simulink model "EsamblajeCohete2_0"  (R2023a)
settings: Solver=VariableStepAuto  StartTime=0.0  StopTime=120  RelTol=1e-3
model workspace: external: MATLAB File C:\Users\SEBASTIANDIAZPABON\OneDrive - Universidad Santo Tomás Bucaramanga\USTA\Semillero Cohete\Cohete Matlab 2.0\EsamblajeCohete2_0_DataFile.m (data not in the file)
undefined symbols (not defined in the file): smiData, X, Y, Z
libraries: sm_lib x354, nesl_utility x13, simulink x7, fuzblock x6
(part 1 of 7)
settings Model: SimulationMode=accelerator  Creator=SEBASTIANDIAZPABON  LastModifiedBy=SEBASTIANDIAZPABON
settings ModelReferenceCC: EnableRefExpFcnMdlSchedulingChecks=on

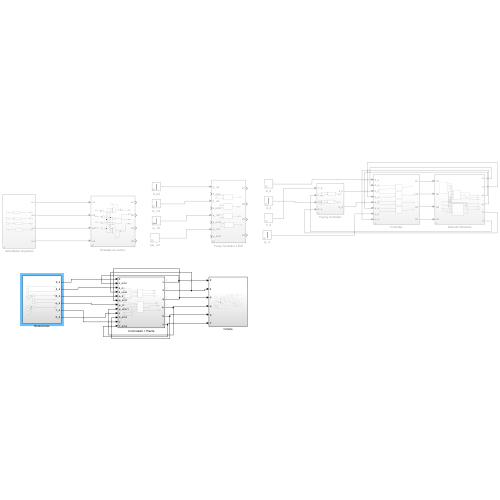
[thumbnail: Simulink's stored preview of the top-level diagram]
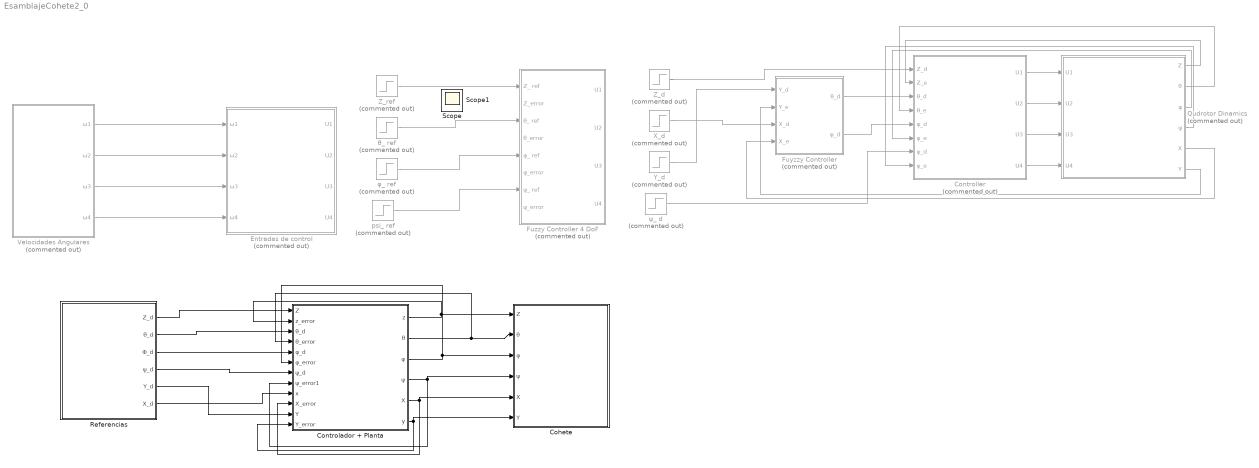
== system EsamblajeCohete2_0 ==
  Cohete : Subsystem
  Controlador + Planta : Subsystem
  Controller : Subsystem  Commented=on
  "Entradas de control " : Subsystem  Commented=on
  Fuyzzy Controller : Subsystem  Commented=on
  Fuzzy Controller 4 DoF : Subsystem  Commented=on
  Qudrotor Dinamics : Subsystem  Commented=on
  Referencias : Subsystem
  Velocidades Angulares : Subsystem  Commented=on
  X_d : Step  Commented=on  After=20  SampleTime=0
  Y_d : Step  Commented=on  After=20  SampleTime=0
  Z_d : Step  Commented=on  Time=0.01  After=30  SampleTime=0
  Z_ref : Step  Commented=on  Time=0  After=0  SampleTime=0
  psi_ ref : Step  Commented=on  Time=0  After=0.05  SampleTime=0
  θ_ ref : Step  Commented=on  Time=0  After=0.1  SampleTime=0
  φ_ ref : Step  Commented=on  Time=0  After=0.5  SampleTime=0
  ψ_ d : Step  Commented=on  After=20  SampleTime=0
  Scope : Scope
  Scope1 : Scope
  wires:
  Velocidades Angulares/1(ω1) -> "Entradas de control "/1(ω1)
  Velocidades Angulares/2(ω2) -> "Entradas de control "/2(ω2)
  Velocidades Angulares/3(ω3) -> "Entradas de control "/3(ω3)
  Velocidades Angulares/4(ω4) -> "Entradas de control "/4(ω4)
  Z_ref/1 -> Fuzzy Controller 4 DoF/1(Z_ ref)
  θ_ ref/1 -> Fuzzy Controller 4 DoF/3(θ_ ref)
  φ_ ref/1 -> Fuzzy Controller 4 DoF/5(φ_ ref)
  psi_ ref/1 -> Fuzzy Controller 4 DoF/7(ψ_ ref)
  Controller/1(U1) -> Qudrotor Dinamics/1(U1)
  Controller/2(U2) -> Qudrotor Dinamics/2(U2)
  Controller/3(U3) -> Qudrotor Dinamics/3(U3)
  Controller/4(U4) -> Qudrotor Dinamics/4(U4)
  Qudrotor Dinamics/1(Z) -> Controller/2(Z_e)
  Qudrotor Dinamics/2(θ) -> Controller/4(θ_e)
  Qudrotor Dinamics/3(φ) -> Controller/6(φ_e)
  Qudrotor Dinamics/4(ψ) -> Controller/8(ψ_e)
  Fuyzzy Controller/1(θ_d) -> Controller/3(θ_d)
  Qudrotor Dinamics/6(Y) -> Fuyzzy Controller/2(Y_e)
  Qudrotor Dinamics/5(X) -> Fuyzzy Controller/4(X_e)
  Fuyzzy Controller/2(φ_d) -> Controller/5(φ_d)
  Z_d/1 -> Controller/1(Z_d)
  X_d/1 -> Fuyzzy Controller/3(X_d)
  Y_d/1 -> Fuyzzy Controller/1(Y_d)
  ψ_ d/1 -> Controller/7(ψ_d)
  Controlador + Planta/1(z) -> Controlador + Planta/2(z_error), Cohete/1(Z)
  Referencias/1(Z_d) -> Controlador + Planta/1(Z)
  Controlador + Planta/2(θ) -> Controlador + Planta/4(θ_error), Cohete/2(θ)
  Controlador + Planta/3(φ) -> Cohete/3(φ), Controlador + Planta/6(φ_error)
  Controlador + Planta/4(ψ) -> Controlador + Planta/8(ψ_error1), Cohete/4(ψ)
  Referencias/2(θ_d) -> Controlador + Planta/3(θ_d)
  Referencias/4(ψ_d) -> Controlador + Planta/7(ψ_d)
  Referencias/3(Φ_d) -> Controlador + Planta/5(φ_d)
  Controlador + Planta/5(X) -> Controlador + Planta/10(X_error), Cohete/5(X)
  Referencias/6(X_d) -> Controlador + Planta/9(x)
  Controlador + Planta/6(y) -> Cohete/6(Y), Controlador + Planta/12(Y_error)
  Referencias/5(Y_d) -> Controlador + Planta/11(Y)

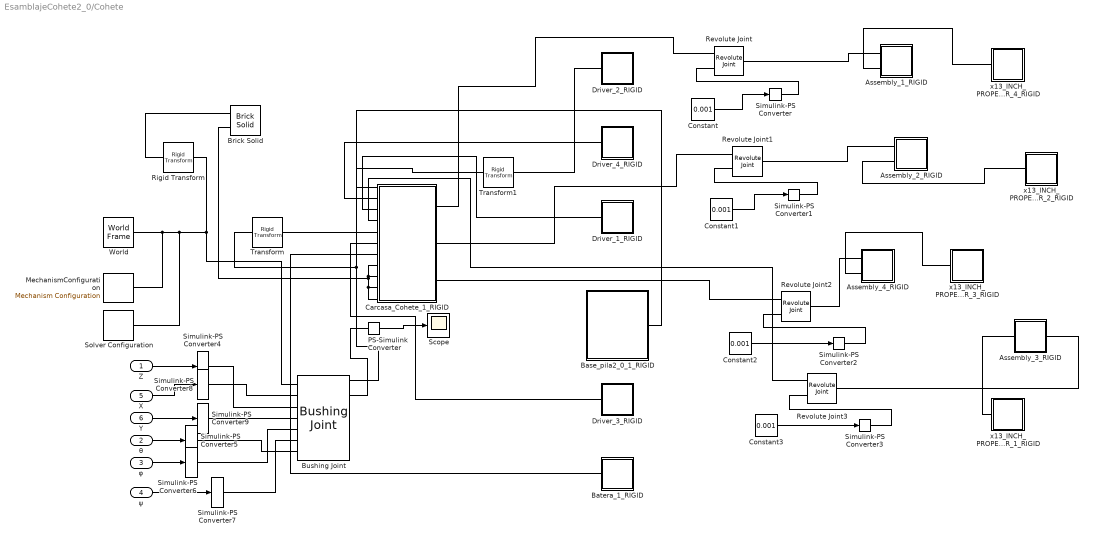
== system EsamblajeCohete2_0/Cohete ==
  Z : Inport
  θ : Inport  Port=2
  φ : Inport  Port=3
  ψ : Inport  Port=4
  X : Inport  Port=5
  Y : Inport  Port=6
  Assembly_1_RIGID : Subsystem
  Assembly_2_RIGID : Subsystem
  Assembly_3_RIGID : Subsystem
  Assembly_4_RIGID : Subsystem
  Base_pila2_0_1_RIGID : Subsystem
  Batera_1_RIGID : Subsystem
  Brick Solid : sm_lib/Body Elements/Brick Solid  GraphicAmbientColor=[0.15 0.15 0.15 1.0]  BasedOnType=Density  BrickDimensions=[2 2 0.1 ]  BrickDimensionsUnits=m  CenterOfMass=[0 0 0]  CenterOfMassUnits=m  GraphicDiffuseColor=[0.4 0.6 0.0]  Density=1000  DensityUnits=kg/m^3  DoExposeReferenceFrame=on  GraphicEmissiveColor=[0.0 0.0 0.0 1.0]  ExportEntireGeometry=on  SerializedFrames=<Frames><Frame><Id>Frame1</Id><Value><Name>F1</Name><Origin><Source>ReferenceFrame</Source><FeatureName></FeatureName></Origin><PrimaryAxis><DefinedDirection>+Y</DefinedDirection><Source>ReferenceFrame</Source><SourceDirection>-Z</SourceDirection><FeatureName></FeatureName></PrimaryAxis><SecondaryAxis><DefinedDirection>+X</DefinedDirection><Source>ReferenceFrame</Source><SourceDirection>+X</SourceDirection><FeatureName></FeatureName></SecondaryAxis></Value></Frame></Frames>  MarkerShape=Sphere  MarkerSize=10  GraphicType=FromGeometry  InertiaType=CalculateFromGeometry  Mass=1  MassUnits=kg  MomentsOfInertia=[1 1 1]  MomentsOfInertiaUnits=kg*m^2  GraphicOpacity=1.0  ProductsOfInertia=[0 0 0]  ProductsOfInertiaUnits=kg*m^2  GraphicShininess=75  GraphicSpecularColor=[0.5 0.5 0.5 1.0]  GraphicVisPropType=SimpleVisualProperties
  Bushing Joint : sm_lib/Joints/Bushing Joint  JointMode=Normal  SenseConstraintForce=off  SenseConstraintForceX=off  SenseConstraintForceY=off  SenseConstraintForceZ=off  SenseConstraintTorque=off  SenseConstraintTorqueX=off  SenseConstraintTorqueY=off  SenseConstraintTorqueZ=off  SenseTotalForce=off  SenseTotalForceX=off  SenseTotalForceY=off  SenseTotalForceZ=off  SenseTotalTorque=off  SenseTotalTorqueX=off  SenseTotalTorqueY=off  SenseTotalTorqueZ=off  CompositeWrenchDir=FollowerOnBase  CompositeWrenchFrame=BaseFrame  PxEquilibriumPosition=0  PxEquilibriumPositionUnits=m  PxSpringStiffness=0  PxSpringStiffnessUnits=N/m  PxDampingCoefficient=0  PxDampingCoefficientUnits=N/(m/s)  PxTorqueActuationMode=ComputedTorque  PxMotionActuationMode=InputMotion  PxSensePosition=off  PxSenseVelocity=off  PxSenseAcceleration=off  PxSenseTorqueForce=on  PxSenseLowerLimitTorqueForce=off  PxSenseUpperLimitTorqueForce=off  PxLowerLimitSpecify=off  PxLowerLimitBound=-1  PxLowerLimitBoundUnits=m  PxLowerLimitStiffness=1e6  PxLowerLimitStiffnessUnits=N/m  PxLowerLimitDamping=1e3  PxLowerLimitDampingUnits=N/(m/s)  PxLowerLimitTransitionRegionWidth=1e-4  PxLowerLimitTransitionRegionWidthUnits=m  PxUpperLimitSpecify=off  PxUpperLimitBound=1  PxUpperLimitBoundUnits=m  PxUpperLimitStiffness=1e6  PxUpperLimitStiffnessUnits=N/m  PxUpperLimitDamping=1e3  PxUpperLimitDampingUnits=N/(m/s)  PxUpperLimitTransitionRegionWidth=1e-4  PxUpperLimitTransitionRegionWidthUnits=m  PxPositionTargetSpecify=off  PxPositionTargetPriority=High  PxPositionTargetValue=0  PxPositionTargetValueUnits=m  PxVelocityTargetSpecify=off  PxVelocityTargetPriority=High  PxVelocityTargetValue=0  PxVelocityTargetValueUnits=m/s  PyEquilibriumPosition=0  PyEquilibriumPositionUnits=m  PySpringStiffness=0  PySpringStiffnessUnits=N/m  PyDampingCoefficient=0  PyDampingCoefficientUnits=N/(m/s)  PyTorqueActuationMode=ComputedTorque  PyMotionActuationMode=InputMotion  PySensePosition=on  PySenseVelocity=on  PySenseAcceleration=off  PySenseTorqueForce=off  PySenseLowerLimitTorqueForce=off  PySenseUpperLimitTorqueForce=off  PyLowerLimitSpecify=off  PyLowerLimitBound=-1  PyLowerLimitBoundUnits=m  PyLowerLimitStiffness=1e6  PyLowerLimitStiffnessUnits=N/m  PyLowerLimitDamping=1e3  PyLowerLimitDampingUnits=N/(m/s)  PyLowerLimitTransitionRegionWidth=1e-4  PyLowerLimitTransitionRegionWidthUnits=m  PyUpperLimitSpecify=off  PyUpperLimitBound=1  PyUpperLimitBoundUnits=m  PyUpperLimitStiffness=1e6  PyUpperLimitStiffnessUnits=N/m  PyUpperLimitDamping=1e3  PyUpperLimitDampingUnits=N/(m/s)  PyUpperLimitTransitionRegionWidth=1e-4  PyUpperLimitTransitionRegionWidthUnits=m  PyPositionTargetSpecify=off  PyPositionTargetPriority=High  PyPositionTargetValue=0  PyPositionTargetValueUnits=m  PyVelocityTargetSpecify=off  PyVelocityTargetPriority=High  PyVelocityTargetValue=0  PyVelocityTargetValueUnits=m/s  PzEquilibriumPosition=0  PzEquilibriumPositionUnits=m  PzSpringStiffness=0  PzSpringStiffnessUnits=N/m  PzDampingCoefficient=0  PzDampingCoefficientUnits=N/(m/s)  PzTorqueActuationMode=ComputedTorque  PzMotionActuationMode=InputMotion  PzSensePosition=off  PzSenseVelocity=off  PzSenseAcceleration=off  PzSenseTorqueForce=off  PzSenseLowerLimitTorqueForce=off  PzSenseUpperLimitTorqueForce=off  PzLowerLimitSpecify=off  PzLowerLimitBound=-1  PzLowerLimitBoundUnits=m  PzLowerLimitStiffness=1e6  PzLowerLimitStiffnessUnits=N/m  PzLowerLimitDamping=1e3  PzLowerLimitDampingUnits=N/(m/s)  PzLowerLimitTransitionRegionWidth=1e-4  PzLowerLimitTransitionRegionWidthUnits=m  PzUpperLimitSpecify=off  PzUpperLimitBound=1  PzUpperLimitBoundUnits=m  PzUpperLimitStiffness=1e6  PzUpperLimitStiffnessUnits=N/m  PzUpperLimitDamping=1e3  PzUpperLimitDampingUnits=N/(m/s)  PzUpperLimitTransitionRegionWidth=1e-4  PzUpperLimitTransitionRegionWidthUnits=m  PzPositionTargetSpecify=off  PzPositionTargetPriority=High  PzPositionTargetValue=0  PzPositionTargetValueUnits=m  PzVelocityTargetSpecify=off  PzVelocityTargetPriority=High  PzVelocityTargetValue=0  PzVelocityTargetValueUnits=m/s  RxEquilibriumPosition=0  RxEquilibriumPositionUnits=deg  RxSpringStiffness=0  RxSpringStiffnessUnits=N*m/deg  RxDampingCoefficient=0  RxDampingCoefficientUnits=N*m/(deg/s)  RxTorqueActuationMode=ComputedTorque  RxMotionActuationMode=InputMotion  RxSensePosition=on  RxSenseVelocity=on  RxSenseAcceleration=off  RxSenseTorqueForce=off  RxSenseLowerLimitTorqueForce=off  RxSenseUpperLimitTorqueForce=off  RxLowerLimitSpecify=off  RxLowerLimitBound=-90  RxLowerLimitBoundUnits=deg  RxLowerLimitStiffness=1e4  RxLowerLimitStiffnessUnits=N*m/deg  RxLowerLimitDamping=10  RxLowerLimitDampingUnits=N*m/(deg/s)  RxLowerLimitTransitionRegionWidth=0.1  RxLowerLimitTransitionRegionWidthUnits=deg  RxUpperLimitSpecify=off  RxUpperLimitBound=90  RxUpperLimitBoundUnits=deg  RxUpperLimitStiffness=1e4  RxUpperLimitStiffnessUnits=N*m/deg  RxUpperLimitDamping=10  RxUpperLimitDampingUnits=N*m/(deg/s)  RxUpperLimitTransitionRegionWidth=0.1  RxUpperLimitTransitionRegionWidthUnits=deg  RxPositionTargetSpecify=off  RxPositionTargetPriority=High  RxPositionTargetValue=0  RxPositionTargetValueUnits=deg  RxVelocityTargetSpecify=off  RxVelocityTargetPriority=High  RxVelocityTargetValue=0  RxVelocityTargetValueUnits=deg/s  RyEquilibriumPosition=0  RyEquilibriumPositionUnits=deg  RySpringStiffness=0  RySpringStiffnessUnits=N*m/deg  RyDampingCoefficient=0  RyDampingCoefficientUnits=N*m/(deg/s)  RyTorqueActuationMode=ComputedTorque  RyMotionActuationMode=InputMotion  RySensePosition=off  RySenseVelocity=off  RySenseAcceleration=off  RySenseTorqueForce=off  RySenseLowerLimitTorqueForce=off  RySenseUpperLimitTorqueForce=off  RyLowerLimitSpecify=off  RyLowerLimitBound=-90  RyLowerLimitBoundUnits=deg  RyLowerLimitStiffness=1e4  RyLowerLimitStiffnessUnits=N*m/deg  RyLowerLimitDamping=10  RyLowerLimitDampingUnits=N*m/(deg/s)  RyLowerLimitTransitionRegionWidth=0.1  RyLowerLimitTransitionRegionWidthUnits=deg  RyUpperLimitSpecify=off  RyUpperLimitBound=90  RyUpperLimitBoundUnits=deg  RyUpperLimitStiffness=1e4  RyUpperLimitStiffnessUnits=N*m/deg  RyUpperLimitDamping=10  RyUpperLimitDampingUnits=N*m/(deg/s)  RyUpperLimitTransitionRegionWidth=0.1  RyUpperLimitTransitionRegionWidthUnits=deg  RyPositionTargetSpecify=off  RyPositionTargetPriority=High  RyPositionTargetValue=0  RyPositionTargetValueUnits=deg  RyVelocityTargetSpecify=off  RyVelocityTargetPriority=High  RyVelocityTargetValue=0  RyVelocityTargetValueUnits=deg/s  RzEquilibriumPosition=0  RzEquilibriumPositionUnits=deg  RzSpringStiffness=0  RzSpringStiffnessUnits=N*m/deg  RzDampingCoefficient=0  RzDampingCoefficientUnits=N*m/(deg/s)  RzTorqueActuationMode=ComputedTorque  RzMotionActuationMode=InputMotion  RzSensePosition=off  RzSenseVelocity=off  RzSenseAcceleration=off  RzSenseTorqueForce=off  RzSenseLowerLimitTorqueForce=off  RzSenseUpperLimitTorqueForce=off  RzLowerLimitSpecify=off  RzLowerLimitBound=-90  RzLowerLimitBoundUnits=deg  RzLowerLimitStiffness=1e4  RzLowerLimitStiffnessUnits=N*m/deg  RzLowerLimitDamping=10  RzLowerLimitDampingUnits=N*m/(deg/s)  RzLowerLimitTransitionRegionWidth=0.1  RzLowerLimitTransitionRegionWidthUnits=deg  RzUpperLimitSpecify=off  RzUpperLimitBound=90  RzUpperLimitBoundUnits=deg  RzUpperLimitStiffness=1e4  RzUpperLimitStiffnessUnits=N*m/deg  RzUpperLimitDamping=10  RzUpperLimitDampingUnits=N*m/(deg/s)  RzUpperLimitTransitionRegionWidth=0.1  RzUpperLimitTransitionRegionWidthUnits=deg  RzPositionTargetSpecify=off  RzPositionTargetPriority=High  RzPositionTargetValue=0  RzPositionTargetValueUnits=deg  RzVelocityTargetSpecify=off  RzVelocityTargetPriority=High  RzVelocityTargetValue=0  RzVelocityTargetValueUnits=deg/s
  Carcasa_Cohete_1_RIGID : Subsystem
  Constant{,1..3} (4 alike) : Constant  Value=0.001
  Driver_1_RIGID : Subsystem
  Driver_2_RIGID : Subsystem
  Driver_3_RIGID : Subsystem
  Driver_4_RIGID : Subsystem
  MechanismConfiguration : sm_lib/Utilities/Mechanism Configuration  UniformGravity=Constant  GravityVector=[0 -9.8 0]  GravityVectorUnits=m/s^2  LinearizationDelta=0.001  JointModeTransitionNonlinearIterations=2
  PS-Simulink Converter : nesl_utility/PS-Simulink Converter  PhysicalDomain=network_engine_domain  SubClassName=ps_output  LeftPortType=input  RightPortType=output  PseudoPeriodic=off  Frequencies=[]  VectorFormat=inherit  Unit=inherit  AffineConversion=off
  Revolute Joint{,1..3} (4 alike) : sm_lib/Joints/Revolute Joint  JointMode=Normal  SenseConstraintForce=off  SenseConstraintForceX=off  SenseConstraintForceY=off  SenseConstraintForceZ=off  SenseConstraintTorque=off  SenseConstraintTorqueX=off  SenseConstraintTorqueY=off  SenseConstraintTorqueZ=off  SenseTotalForce=off  SenseTotalForceX=off  SenseTotalForceY=off  SenseTotalForceZ=off  SenseTotalTorque=off  SenseTotalTorqueX=off  SenseTotalTorqueY=off  SenseTotalTorqueZ=off  CompositeWrenchDir=FollowerOnBase  CompositeWrenchFrame=BaseFrame  EquilibriumPosition=0  EquilibriumPositionUnits=deg  SpringStiffness=0  SpringStiffnessUnits=N*m/deg  DampingCoefficient=0  DampingCoefficientUnits=N*m/(deg/s)  TorqueActuationMode=InputTorque  MotionActuationMode=ComputedMotion  SensePosition=off  SenseVelocity=off  SenseAcceleration=off  SenseTorqueForce=off  SenseLowerLimitTorqueForce=off  SenseUpperLimitTorqueForce=off  LowerLimitSpecify=off  LowerLimitBound=-90  LowerLimitBoundUnits=deg  LowerLimitStiffness=1e4  LowerLimitStiffnessUnits=N*m/deg  LowerLimitDamping=10  LowerLimitDampingUnits=N*m/(deg/s)  LowerLimitTransitionRegionWidth=0.1  LowerLimitTransitionRegionWidthUnits=deg  UpperLimitSpecify=off  UpperLimitBound=90  UpperLimitBoundUnits=deg  UpperLimitStiffness=1e4  UpperLimitStiffnessUnits=N*m/deg  UpperLimitDamping=10  UpperLimitDampingUnits=N*m/(deg/s)  UpperLimitTransitionRegionWidth=0.1  UpperLimitTransitionRegionWidthUnits=deg  PositionTargetSpecify=off  PositionTargetPriority=High  PositionTargetValue=0  PositionTargetValueUnits=deg  VelocityTargetSpecify=off  VelocityTargetPriority=High  VelocityTargetValue=0  VelocityTargetValueUnits=deg/s
  Rigid Transform : sm_lib/Frames and Transforms/Rigid Transform  TranslationMethod=Cartesian  TranslationStandardOffset=0  TranslationStandardOffsetUnits=m  TranslationStandardAxis=+Z  TranslationCartesianOffset=[0 0.182 0]  TranslationCartesianOffsetUnits=m  TranslationROffset=0  TranslationROffsetUnits=m  TranslationZOffset=0  TranslationZOffsetUnits=m  TranslationThetaOffset=0  TranslationThetaOffsetUnits=deg  RotationMethod=None  RotationAngleUnits=deg  RotationStandardAxis=+Z  RotationAngle=0.0  RotationArbitraryAxis=[0 0 1]  FollAlignAxisA=+X  BaseAlignAxisA=+Y  FollAlignAxisB=+Y  BaseAlignAxisB=+Z  RotationSequenceAxes=FollowerAxes  RotationSequence=XYX  RotationSequenceAngles=[0 0 0]  RotationSequenceAnglesUnits=deg  RotationMatrix=[1 0 0; 0 1 0; 0 0 1]  Quaternion=[1 0 0 0]
  Scope : Scope
  Simulink-PS Converter{,1..3} (4 alike) : nesl_utility/Simulink-PS Converter  PhysicalDomain=network_engine_domain  SubClassName=ps_input  LeftPortType=input  RightPortType=output  PseudoPeriodic=off  Frequencies=[]  NoiseDistribution=none  NoiseParameters=[]  Unit=1  AffineConversion=off  FilteringAndDerivatives=provide  SimscapeFilterOrder=1  InputFilterTimeConstant=0.001  UdotUserProvided=0
  Simulink-PS Converter{4..9} (6 alike) : nesl_utility/Simulink-PS Converter  PhysicalDomain=network_engine_domain  SubClassName=ps_input  LeftPortType=input  RightPortType=output  PseudoPeriodic=off  Frequencies=[]  NoiseDistribution=none  NoiseParameters=[]  Unit=1  AffineConversion=off  FilteringAndDerivatives=filter  SimscapeFilterOrder=2  InputFilterTimeConstant=0.001  UdotUserProvided=0
  Solver Configuration : nesl_utility/Solver Configuration  PhysicalDomain=network_engine_domain  SubClassName=solver  LeftPortType=input  RightPortType=generic  Tones=[]  Harmonics=[]  SimulateNoise=off  Profile=off  UseLocalSampling=off  EnableSwitchedLinearOptims=on  FrequencyDomain=off  UseCCode=off  RelTol=0.001  AbsTol=0.001  MinStep=1e-09  ToWorkspace=off  RevertToSquareIcSolve=off  NumHomotopyIterations=100  PhasorMode=off  PhasorModeNumHarmonics=1  ConsistencySolver=NEWTON_FTOL  IndexReductionMethod=DerivativeReplacement  DoDC=off  ResidualTolerance=1e-09  ConsistencyTolSource=GLOBAL  ConsistencyAbsTol=0.001  ConsistencyRelTol=0.001  ConsistencyTolFactor=0.001  UseLocalSolver=off  LocalSolverChoice=NE_BACKWARD_EULER_ADVANCER  ResolveIndetEquations=on  FunctionEvalNumThread=1  LocalSolverSampleTime=0.001  DoFixedCost=off  MaxNonlinIter=3  MaxModeIter=2  ComputeImpulses=off  ImpulseIterations=2  LinearAlgebra=auto  LinearAlgebraNumThread=0  EquationFormulation=NE_TIME_EF  DelaysMemoryBudget=1024  AutomaticFiltering=on  FilteringTimeConstant=0.001  PartitionStorageMethod=AS_NEEDED  PartitionMemoryBudget=1024  PartitionMethod=ROBUST
  Transform : sm_lib/Frames and Transforms/Rigid Transform  TranslationMethod=Cartesian  TranslationStandardOffset=0  TranslationStandardOffsetUnits=mm  TranslationStandardAxis=+Z  TranslationCartesianOffset=smiData.RigidTransform(12).translation  TranslationCartesianOffsetUnits=mm  TranslationROffset=0  TranslationROffsetUnits=m  TranslationZOffset=0  TranslationZOffsetUnits=m  TranslationThetaOffset=0  TranslationThetaOffsetUnits=deg  RotationMethod=ArbitraryAxis  RotationAngleUnits=rad  RotationStandardAxis=+Z  RotationAngle=smiData.RigidTransform(12).angle  RotationArbitraryAxis=smiData.RigidTransform(12).axis  FollAlignAxisA=+X  BaseAlignAxisA=+Y  FollAlignAxisB=+Y  BaseAlignAxisB=+Z  RotationSequenceAxes=FollowerAxes  RotationSequence=XYX  RotationSequenceAngles=[0 0 0]  RotationSequenceAnglesUnits=deg  RotationMatrix=[1 0 0; 0 1 0; 0 0 1]  Quaternion=[1 0 0 0]
  Transform1 : sm_lib/Frames and Transforms/Rigid Transform  TranslationMethod=Cartesian  TranslationStandardOffset=0  TranslationStandardOffsetUnits=mm  TranslationStandardAxis=+Z  TranslationCartesianOffset=smiData.RigidTransform(123).translation  TranslationCartesianOffsetUnits=mm  TranslationROffset=0  TranslationROffsetUnits=m  TranslationZOffset=0  TranslationZOffsetUnits=m  TranslationThetaOffset=0  TranslationThetaOffsetUnits=deg  RotationMethod=ArbitraryAxis  RotationAngleUnits=rad  RotationStandardAxis=+Z  RotationAngle=smiData.RigidTransform(123).angle  RotationArbitraryAxis=smiData.RigidTransform(123).axis  FollAlignAxisA=+X  BaseAlignAxisA=+Y  FollAlignAxisB=+Y  BaseAlignAxisB=+Z  RotationSequenceAxes=FollowerAxes  RotationSequence=XYX  RotationSequenceAngles=[0 0 0]  RotationSequenceAnglesUnits=deg  RotationMatrix=[1 0 0; 0 1 0; 0 0 1]  Quaternion=[1 0 0 0]
  World : sm_lib/Frames and Transforms/World Frame
  x13_INCH_PROPELLER_1_RIGID : Subsystem
  x13_INCH_PROPELLER_2_RIGID : Subsystem
  x13_INCH_PROPELLER_3_RIGID : Subsystem
  x13_INCH_PROPELLER_4_RIGID : Subsystem
  wires:
  θ/1 -> Simulink-PS Converter5/1
  φ/1 -> Simulink-PS Converter6/1
  ψ/1 -> Simulink-PS Converter7/1
  Z/1 -> Simulink-PS Converter4/1
  X/1 -> Simulink-PS Converter8/1
  Y/1 -> Simulink-PS Converter9/1
  Constant/1 -> Simulink-PS Converter/1
  Constant1/1 -> Simulink-PS Converter1/1
  Constant2/1 -> Simulink-PS Converter2/1
  Constant3/1 -> Simulink-PS Converter3/1
  PS-Simulink Converter/1 -> Scope/1
  connections:
  Driver_2_RIGID/LConn1 -- Transform1/RConn1
  Assembly_3_RIGID/LConn1 -- x13_INCH_PROPELLER_1_RIGID/LConn1
  Transform/RConn1 -- Carcasa_Cohete_1_RIGID/LConn5
  Base_pila2_0_1_RIGID/RConn1 -- Carcasa_Cohete_1_RIGID/LConn1
  Assembly_4_RIGID/LConn2 -- x13_INCH_PROPELLER_3_RIGID/LConn1
  Transform1/LConn1 -- Bushing Joint/RConn1 -- Transform/LConn1
  Batera_1_RIGID/LConn1 -- Carcasa_Cohete_1_RIGID/LConn7
  Assembly_1_RIGID/LConn2 -- x13_INCH_PROPELLER_4_RIGID/LConn1
  Driver_4_RIGID/LConn1 -- Carcasa_Cohete_1_RIGID/LConn2
  Driver_3_RIGID/LConn1 -- Carcasa_Cohete_1_RIGID/LConn6
  Driver_1_RIGID/LConn1 -- Carcasa_Cohete_1_RIGID/LConn3
  Assembly_2_RIGID/LConn2 -- x13_INCH_PROPELLER_2_RIGID/LConn1
  Brick Solid/LConn2 -- Carcasa_Cohete_1_RIGID/LConn8 -- Carcasa_Cohete_1_RIGID/LConn9 -- Carcasa_Cohete_1_RIGID/LConn11 -- Carcasa_Cohete_1_RIGID/LConn10
  Carcasa_Cohete_1_RIGID/RConn2 -- Revolute Joint1/LConn1
  Carcasa_Cohete_1_RIGID/RConn1 -- Revolute Joint/LConn1
  Revolute Joint2/RConn1 -- Assembly_4_RIGID/LConn1
  Carcasa_Cohete_1_RIGID/LConn4 -- Revolute Joint3/LConn1
  MechanismConfiguration/RConn1 -- World/RConn1 -- Bushing Joint/LConn1 -- Rigid Transform/RConn1 -- Solver Configuration/RConn1
  Rigid Transform/LConn1 -- Brick Solid/LConn1
  Simulink-PS Converter4/RConn1 -- Bushing Joint/LConn3
  Simulink-PS Converter5/RConn1 -- Bushing Joint/LConn7
  Simulink-PS Converter6/RConn1 -- Bushing Joint/LConn5
  Simulink-PS Converter7/RConn1 -- Bushing Joint/LConn6
  Simulink-PS Converter8/RConn1 -- Bushing Joint/LConn2
  Bushing Joint/LConn4 -- Simulink-PS Converter9/RConn1
  Revolute Joint/RConn1 -- Assembly_1_RIGID/LConn1
  Simulink-PS Converter/RConn1 -- Revolute Joint/LConn2
  Revolute Joint1/LConn2 -- Simulink-PS Converter1/RConn1
  Revolute Joint1/RConn1 -- Assembly_2_RIGID/LConn1
  Simulink-PS Converter2/RConn1 -- Revolute Joint2/LConn2
  Revolute Joint2/LConn1 -- Carcasa_Cohete_1_RIGID/RConn3
  Simulink-PS Converter3/RConn1 -- Revolute Joint3/LConn2
  Revolute Joint3/RConn1 -- Assembly_3_RIGID/RConn1
  PS-Simulink Converter/LConn1 -- Bushing Joint/RConn2

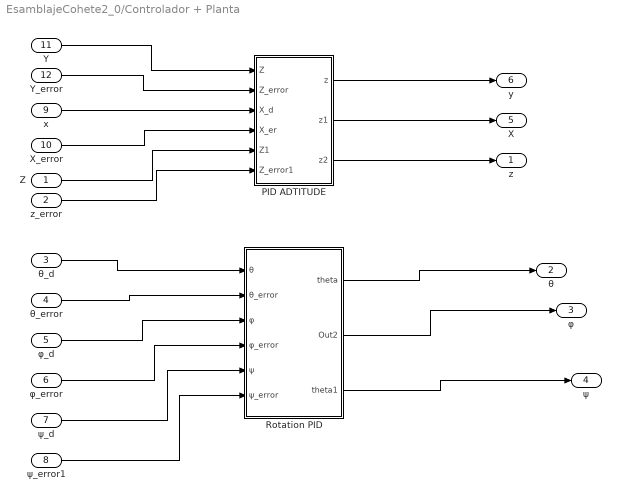
== system EsamblajeCohete2_0/Controlador + Planta ==
  Z : Inport
  z_error : Inport  Port=2
  θ_d : Inport  Port=3
  θ_error : Inport  Port=4
  φ_d : Inport  Port=5
  φ_error : Inport  Port=6
  ψ_d : Inport  Port=7
  ψ_error1 : Inport  Port=8
  x : Inport  Port=9
  X_error : Inport  Port=10
  Y : Inport  Port=11
  Y_error : Inport  Port=12
  PID ADTITUDE : Subsystem
  Rotation PID : Subsystem
  z : Outport
  θ : Outport  Port=2
  φ : Outport  Port=3
  ψ : Outport  Port=4
  X : Outport  Port=5
  y : Outport  Port=6
  wires:
  Y/1 -> PID ADTITUDE/1(Z)
  Y_error/1 -> PID ADTITUDE/2(Z_error)
  x/1 -> PID ADTITUDE/3(X_d)
  X_error/1 -> PID ADTITUDE/4(X_er)
  Z/1 -> PID ADTITUDE/5(Z1)
  z_error/1 -> PID ADTITUDE/6(Z_error1)
  PID ADTITUDE/1(z) -> y/1
  PID ADTITUDE/2(z1) -> X/1
  PID ADTITUDE/3(z2) -> z/1
  θ_d/1 -> Rotation PID/1(θ)
  θ_error/1 -> Rotation PID/2(θ_error)
  φ_d/1 -> Rotation PID/3(φ)
  φ_error/1 -> Rotation PID/4(φ_error)
  ψ_d/1 -> Rotation PID/5(ψ)
  ψ_error1/1 -> Rotation PID/6(ψ_error)
  Rotation PID/1(theta) -> θ/1
  Rotation PID/2(Out2) -> φ/1
  Rotation PID/3(theta1) -> ψ/1

== system EsamblajeCohete2_0/Controller ==
  Z_d : Inport
  Z_e : Inport  Port=2
  θ_d : Inport  Port=3
  θ_e : Inport  Port=4
  φ_d : Inport  Port=5
  φ_e : Inport  Port=6
  ψ_d : Inport  Port=7
  ψ_e : Inport  Port=8
  PID ATITUDE : Subsystem
  "PID θ   " : Subsystem
  PID φ : Subsystem
  PID ψ : Subsystem
  U1 : Outport
  U2 : Outport  Port=2
  U3 : Outport  Port=3
  U4 : Outport  Port=4
  wires:
  PID ATITUDE/1(U1) -> U1/1
  "PID θ   "/1(U2) -> U2/1
  Z_d/1 -> PID ATITUDE/1(Z)
  Z_e/1 -> PID ATITUDE/2(Z_error)
  θ_d/1 -> "PID θ   "/1(θ)
  θ_e/1 -> "PID θ   "/2(θ_error)
  φ_d/1 -> PID φ/1(φ)
  φ_e/1 -> PID φ/2(φ_error)
  PID φ/1(U3) -> U3/1
  PID ψ/1(U4) -> U4/1
  ψ_d/1 -> PID ψ/1(ψ)
  ψ_e/1 -> PID ψ/2(ψ_error)

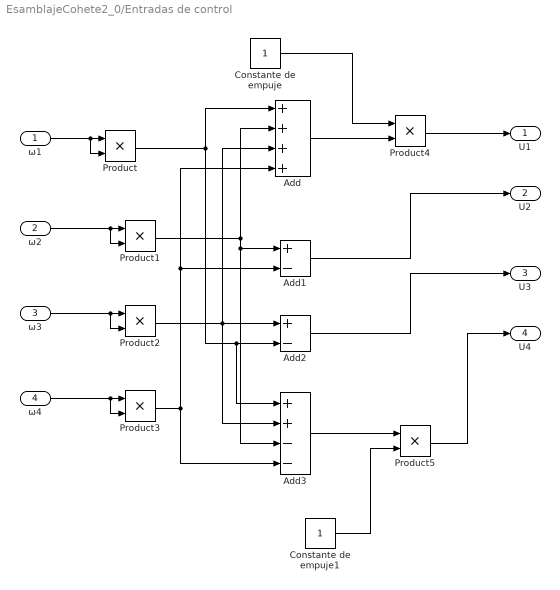
== system EsamblajeCohete2_0/Entradas de control  ==
  ω1 : Inport
  ω2 : Inport  Port=2
  ω3 : Inport  Port=3
  ω4 : Inport  Port=4
  Add : Sum  Inputs=++++
  Add1 : Sum  Inputs=+-
  Add2 : Sum  Inputs=+-
  Add3 : Sum  Inputs=++--
  Constante de empuje : Constant
  Constante de empuje1 : Constant
  Product{,1..5} (6 alike) : Product
  U1 : Outport
  U2 : Outport  Port=2
  U3 : Outport  Port=3
  U4 : Outport  Port=4
  wires:
  ω1/1 -> Product/2, Product/1
  ω2/1 -> Product1/2, Product1/1
  ω3/1 -> Product2/2, Product2/1
  ω4/1 -> Product3/2, Product3/1
  Product/1 -> Add3/1, Add2/2, Add/1
  Product1/1 -> Add1/1, Add3/3, Add/2
  Product2/1 -> Add2/1, Add/3, Add3/2
  Product3/1 -> Add3/4, Add1/2, Add/4
  Add/1 -> Product4/2
  Constante de empuje/1 -> Product4/1
  Product4/1 -> U1/1
  Add1/1 -> U2/1
  Add2/1 -> U3/1
  Add3/1 -> Product5/1
  Constante de empuje1/1 -> Product5/2
  Product5/1 -> U4/1

== system EsamblajeCohete2_0/Fuyzzy Controller ==
  Y_d : Inport
  Y_e : Inport  Port=2
  X_d : Inport  Port=3
  X_e : Inport  Port=4
  Fuzzy Lateral Controller : Subsystem
  Fuzzy Longitudinal Controller : Subsystem
  θ_d : Outport
  φ_d : Outport  Port=2
  wires:
  Y_d/1 -> Fuzzy Longitudinal Controller/1(Y_d)
  Fuzzy Longitudinal Controller/1(θ_d) -> θ_d/1
  Y_e/1 -> Fuzzy Longitudinal Controller/2(Y_e)
  X_d/1 -> Fuzzy Lateral Controller/1(X_d)
  Fuzzy Lateral Controller/1(θ_d) -> φ_d/1
  X_e/1 -> Fuzzy Lateral Controller/2(X_e)

== system EsamblajeCohete2_0/Fuzzy Controller 4 DoF ==
  Z_ ref : Inport
  Z_error : Inport  Port=2
  θ_ ref : Inport  Port=3
  θ_error : Inport  Port=4
  φ_ ref : Inport  Port=5
  φ_error : Inport  Port=6
  ψ_ ref : Inport  Port=7
  ψ_error : Inport  Port=8
  Fuzzy Controller Z : Subsystem
  Fuzzy Controller θ : Subsystem
  Fuzzy Controller φ : Subsystem
  Fuzzy Controller ψ : Subsystem
  U1 : Outport
  U2 : Outport  Port=2
  U3 : Outport  Port=3
  U4 : Outport  Port=4
  wires:
  ψ_ ref/1 -> Fuzzy Controller ψ/1(ψ_ ref)
  θ_error/1 -> Fuzzy Controller θ/2(θ_error)
  ψ_error/1 -> Fuzzy Controller ψ/2(ψ_error)
  φ_error/1 -> Fuzzy Controller φ/2(φ_error)
  θ_ ref/1 -> Fuzzy Controller θ/1(θ_ ref)
  Fuzzy Controller ψ/1(U4) -> U4/1
  φ_ ref/1 -> Fuzzy Controller φ/1(φ_ ref)
  Z_ ref/1 -> Fuzzy Controller Z/1(Z_ ref)
  Z_error/1 -> Fuzzy Controller Z/2(Z_error)
  Fuzzy Controller Z/1(U1) -> U1/1
  Fuzzy Controller θ/1(U3) -> U3/1
  Fuzzy Controller φ/1(U2) -> U2/1

== system EsamblajeCohete2_0/Qudrotor Dinamics ==
  U1 : Inport
  U2 : Inport  Port=2
  U3 : Inport  Port=3
  U4 : Inport  Port=4
  Constantes : Subsystem
  Rotacional : Subsystem
  Traslacional : Subsystem
  Z : Outport
  θ : Outport  Port=2
  φ : Outport  Port=3
  ψ : Outport  Port=4
  X : Outport  Port=5
  Y : Outport  Port=6
  wires:
  Constantes/2(g) -> Traslacional/1(g)
  Constantes/3(m) -> Traslacional/3(m)
  U1/1 -> Traslacional/2(U1)
  Traslacional/1(Z) -> Z/1
  Constantes/4(Ixx) -> Rotacional/1(Ixx)
  Constantes/5(Iyy) -> Rotacional/2(Iyy)
  Constantes/6(Izz) -> Rotacional/3(Izz)
  Constantes/1(l) -> Rotacional/7(L)
  U2/1 -> Rotacional/4(U2)
  U3/1 -> Rotacional/5(U3)
  U4/1 -> Rotacional/6(U4)
  Rotacional/1(θ) -> Traslacional/4(θ), θ/1
  Rotacional/2(φ) -> Traslacional/6(φ), φ/1
  Rotacional/3(ψ) -> Traslacional/5(ψ), ψ/1
  Traslacional/2(X) -> X/1
  Traslacional/3(Y) -> Y/1

== system EsamblajeCohete2_0/Referencias ==
  Add1 : Sum  Inputs=++-
  Add2 : Sum  Inputs=+-
  Ramp1 : simulink/Sources/Ramp  slope=0.017  start=60  InitialOutput=0
  Ramp2 : simulink/Sources/Ramp  slope=1  start=0  InitialOutput=0
  Ramp3 : simulink/Sources/Ramp  slope=1  start=40  InitialOutput=0
  Step1 : Step  After=0.01  SampleTime=0
  Step2 : Step  Time=0.5  After=0.01  SampleTime=0
  Step3 : Step  Time=30  After=0  SampleTime=0
  Step4 : Step  Time=0  After=0  SampleTime=0
  Step5 : Step  After=0  SampleTime=0
  Step6 : Step  SampleTime=0
  Z_d : Outport
  θ_d : Outport  Port=2
  Φ_d : Outport  Port=3
  ψ_d : Outport  Port=4
  Y_d : Outport  Port=5
  X_d : Outport  Port=6
  wires:
  Add1/1 -> ψ_d/1
  Step1/1 -> θ_d/1
  Step2/1 -> Φ_d/1
  Step3/1 -> Add1/2
  Ramp2/1 -> Add1/1
  Ramp3/1 -> Add1/3
  Step4/1 -> Y_d/1
  Step5/1 -> X_d/1
  Add2/1 -> Z_d/1
  Step6/1 -> Add2/1
  Ramp1/1 -> Add2/2

== system EsamblajeCohete2_0/Velocidades Angulares ==
  Step{,1..3} (4 alike) : Step  Time=0.12  After=5  SampleTime=0
  Transfer Fcn{,1..3} (4 alike) : TransferFcn  Numerator=[0.15]  Denominator=[0.0000023 0.0001 0.002683]
  ω1 : Outport
  ω2 : Outport  Port=2
  ω3 : Outport  Port=3
  ω4 : Outport  Port=4
  wires:
  Transfer Fcn/1 -> ω1/1
  Transfer Fcn1/1 -> ω2/1
  Transfer Fcn2/1 -> ω3/1
  Transfer Fcn3/1 -> ω4/1
  Step/1 -> Transfer Fcn/1
  Step1/1 -> Transfer Fcn1/1
  Step2/1 -> Transfer Fcn2/1
  Step3/1 -> Transfer Fcn3/1
